simulink model "2.LC vs. LCL"  (R2022b)
settings: Solver=ode23tb  StartTime=0.0  StopTime=0.06  RelTol=1e-3
libraries: spsCurrentMeasurementLib x18, spsSeriesRLCBranchLib x17, spsIGBTDiodeLib x12, spsabctodq0Lib x4, spsDCVoltageSourceLib x2, spsGroundLib x2, spsThreePhaseSeriesRLCLoadLib x2, spsThreePhaseTransformerTwoWindingsLib x2, spsThreePhaseVIMeasurementLib x2, spsSVPWMGenerator2LevelLib x1, spsabctoAlphaBetaZeroLib x1, spspowerguiLib x1
settings Model: Creator=Mushrif  LastModifiedBy=Mushrif

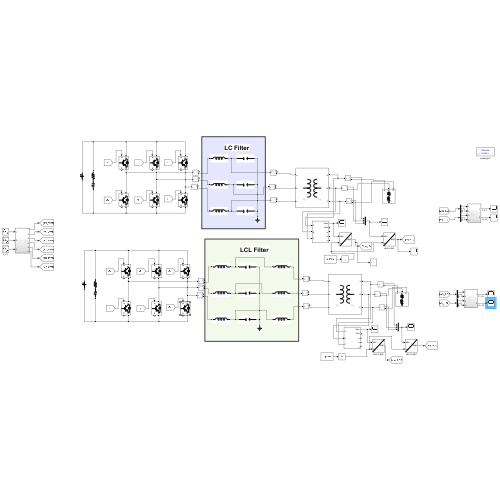
[thumbnail: Simulink's stored preview of the top-level diagram]
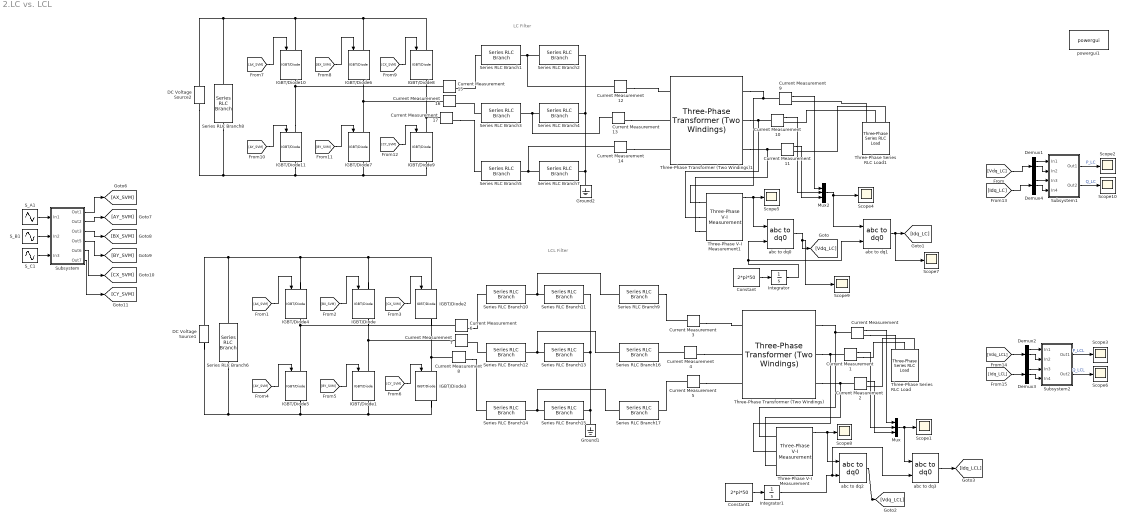
== system 2.LC vs. LCL ==
  note: LCL Filter
  note: LC Filter
  Constant : Constant  Value=2*pi*50
  Constant1 : Constant  Value=2*pi*50
  Current Measurement{,1..17} (18 alike) : spsCurrentMeasurementLib/Current Measurement  PhasorSimulation=off  OutputType=Complex  PSBequivalent=0
  DC Voltage Source1 : spsDCVoltageSourceLib/DC Voltage Source  Amplitude=78  Measurements=None
  DC Voltage Source2 : spsDCVoltageSourceLib/DC Voltage Source  Amplitude=82  Measurements=None
  Demux{1..4} (4 alike) : Demux  Outputs=3
  Ground1 : spsGroundLib/Ground  LConnTagsString=a
  Ground2 : spsGroundLib/Ground  LConnTagsString=a
  IGBT/Diode{,1..11} (12 alike) : spsIGBTDiodeLib/IGBT//Diode  Ron=1e-3  Rs=1e5  Cs=inf  Measurements=on
  Integrator : Integrator
  Integrator1 : Integrator
  Mux : Mux  Inputs=3
  Mux2 : Mux  Inputs=3
  S_A1 : Sin  Amplitude=0.9  Frequency=2*pi*50  SampleTime=0
  S_B1 : Sin  Amplitude=0.9  Frequency=2*pi*50  Phase=-2*pi/3  SampleTime=0
  S_C1 : Sin  Amplitude=0.9  Frequency=2*pi*50  Phase=2*pi/3  SampleTime=0
  Scope{1..10} (10 alike) : Scope
  Series RLC Branch{1,3,5,9,16..17} (6 alike) : spsSeriesRLCBranchLib/Series RLC Branch  LConnTagsString=__new0  RConnTagsString=__new0  BranchType=L  Resistance=2.2  Inductance=250e-6  SetiL0=off  InitialCurrent=0  Capacitance=1e-6  Setx0=off  InitialVoltage=0  Measurements=None
  Series RLC Branch10 : spsSeriesRLCBranchLib/Series RLC Branch  LConnTagsString=__new0  RConnTagsString=__new0  BranchType=L  Resistance=2.2  Inductance=100e-9  SetiL0=off  InitialCurrent=0  Capacitance=1e-6  Setx0=off  InitialVoltage=0  Measurements=None
  Series RLC Branch11 : spsSeriesRLCBranchLib/Series RLC Branch  LConnTagsString=__new0  RConnTagsString=__new0  BranchType=C  Resistance=1  Inductance=1e-3  SetiL0=off  InitialCurrent=0  Capacitance=40e-3  Setx0=off  InitialVoltage=0  Measurements=None
  Series RLC Branch12 : spsSeriesRLCBranchLib/Series RLC Branch  LConnTagsString=__new0  RConnTagsString=__new0  BranchType=L  Resistance=2.2  Inductance=100e-9  SetiL0=off  InitialCurrent=0  Capacitance=1e-6  Setx0=off  InitialVoltage=0  Measurements=None
  Series RLC Branch13 : spsSeriesRLCBranchLib/Series RLC Branch  LConnTagsString=__new0  RConnTagsString=__new0  BranchType=C  Resistance=1  Inductance=1e-3  SetiL0=off  InitialCurrent=0  Capacitance=40e-3  Setx0=off  InitialVoltage=0  Measurements=None
  Series RLC Branch14 : spsSeriesRLCBranchLib/Series RLC Branch  LConnTagsString=__new0  RConnTagsString=__new0  BranchType=L  Resistance=2.2  Inductance=100e-9  SetiL0=off  InitialCurrent=0  Capacitance=1e-6  Setx0=off  InitialVoltage=0  Measurements=None
  Series RLC Branch15 : spsSeriesRLCBranchLib/Series RLC Branch  LConnTagsString=__new0  RConnTagsString=__new0  BranchType=C  Resistance=1  Inductance=1e-3  SetiL0=off  InitialCurrent=0  Capacitance=40e-3  Setx0=off  InitialVoltage=0  Measurements=None
  Series RLC Branch2 : spsSeriesRLCBranchLib/Series RLC Branch  LConnTagsString=__new0  RConnTagsString=__new0  BranchType=C  Resistance=1  Inductance=1e-3  SetiL0=off  InitialCurrent=0  Capacitance=40e-6  Setx0=off  InitialVoltage=0  Measurements=None
  Series RLC Branch4 : spsSeriesRLCBranchLib/Series RLC Branch  LConnTagsString=__new0  RConnTagsString=__new0  BranchType=C  Resistance=1  Inductance=1e-3  SetiL0=off  InitialCurrent=0  Capacitance=40e-6  Setx0=off  InitialVoltage=0  Measurements=None
  Series RLC Branch6 : spsSeriesRLCBranchLib/Series RLC Branch  LConnTagsString=__new0  RConnTagsString=__new0  BranchType=RC  Resistance=0.02  Inductance=1e-3  SetiL0=off  InitialCurrent=0  Capacitance=0.001  Setx0=off  InitialVoltage=0  Measurements=None
  Series RLC Branch7 : spsSeriesRLCBranchLib/Series RLC Branch  LConnTagsString=__new0  RConnTagsString=__new0  BranchType=C  Resistance=1  Inductance=1e-3  SetiL0=off  InitialCurrent=0  Capacitance=40e-6  Setx0=off  InitialVoltage=0  Measurements=None
  Series RLC Branch8 : spsSeriesRLCBranchLib/Series RLC Branch  LConnTagsString=__new0  RConnTagsString=__new0  BranchType=RC  Resistance=0.02  Inductance=1e-3  SetiL0=off  InitialCurrent=0  Capacitance=0.001  Setx0=off  InitialVoltage=0  Measurements=None
  Subsystem : Subsystem
  Subsystem1 : Subsystem
  Subsystem2 : Subsystem
  Three-Phase Series RLC Load : spsThreePhaseSeriesRLCLoadLib/Three-Phase Series RLC Load  LConnTagsString=A|B|C  Configuration=Y (grounded)  NominalVoltage=400  Vabc=[1e3 1e3 1e3]  Vabcp=[1e3 1e3 1e3]  NominalFrequency=50  UnbalancedPower=off  ActivePower=1500  InductivePower=100  CapacitivePower=0  Pabc=[10e3 9e3 11e3]  QLabc=[100 90 110]  QCabc=[100 90 110]  Pabcp=[10e3 9e3 11e3]  QLabcp=[100 90 110]  QCabcp=[100 90 110]  Measurements=None  LoadType=constant Z
  Three-Phase Series RLC Load1 : spsThreePhaseSeriesRLCLoadLib/Three-Phase Series RLC Load  LConnTagsString=A|B|C  Configuration=Y (grounded)  NominalVoltage=400  Vabc=[1e3 1e3 1e3]  Vabcp=[1e3 1e3 1e3]  NominalFrequency=50  UnbalancedPower=off  ActivePower=1500  InductivePower=100  CapacitivePower=0  Pabc=[10e3 9e3 11e3]  QLabc=[100 90 110]  QCabc=[100 90 110]  Pabcp=[10e3 9e3 11e3]  QLabcp=[100 90 110]  QCabcp=[100 90 110]  Measurements=None  LoadType=constant Z
  Three-Phase Transformer (Two Windings) : spsThreePhaseTransformerTwoWindingsLib/Three-Phase Transformer (Two Windings)  Winding1Connection=Yg  Winding2Connection=Yg  CoreType=Three single-phase transformers  SetSaturation=off  Hysteresis=off  DataFile='hysteresis'  SetInitialFlux=off  Measurements=None  UNITS=SI  NominalPower=[ 1900 , 50 ]  Winding1=[415 0.0001 0.0001]  Winding2=[47 0.0001 0.0001]  Rm=45322  Lm=144.27  L0=0.5  Saturation=[0 0;0.0089716 1.2943;3.7382 1.6394]  InitialFluxes=[ 0.8 , -0.8 , 0.7 ]  BreakLoop=off  DiscreteSolver=Trapezoidal iterative  DataType=on  TransfoNumber=1
  Three-Phase Transformer (Two Windings)1 : spsThreePhaseTransformerTwoWindingsLib/Three-Phase Transformer (Two Windings)  Winding1Connection=Yg  Winding2Connection=Yg  CoreType=Three single-phase transformers  SetSaturation=off  Hysteresis=off  DataFile='hysteresis'  SetInitialFlux=off  Measurements=None  UNITS=SI  NominalPower=[ 1900 , 50 ]  Winding1=[415 0.0001 0.0001]  Winding2=[47 0.0001 0.0001]  Rm=45322  Lm=144.27  L0=0.5  Saturation=[0 0;0.0089716 1.2943;3.7382 1.6394]  InitialFluxes=[ 0.8 , -0.8 , 0.7 ]  BreakLoop=off  DiscreteSolver=Trapezoidal iterative  DataType=on  TransfoNumber=1
  Three-Phase V-I Measurement : spsThreePhaseVIMeasurementLib/Three-Phase V-I Measurement  VoltageMeasurement=phase-to-phase  SetLabelV=off  LabelV=Vabc  Vpu=off  VpuLL=off  CurrentMeasurement=yes  SetLabelI=off  LabelI=Iabc  Ipu=off  Pbase=100e6  Vbase=500e3  OutputType=Complex  PhasorSimulation=off  PSBequivalent=0
  Three-Phase V-I Measurement1 : spsThreePhaseVIMeasurementLib/Three-Phase V-I Measurement  VoltageMeasurement=phase-to-phase  SetLabelV=off  LabelV=Vabc  Vpu=off  VpuLL=off  CurrentMeasurement=yes  SetLabelI=off  LabelI=Iabc  Ipu=off  Pbase=100e6  Vbase=500e3  OutputType=Complex  PhasorSimulation=off  PSBequivalent=0
  abc to dq{0..3} (4 alike) : spsabctodq0Lib/abc to dq0  Alignment=90 degrees behind phase A axis
  powergui1 : spspowerguiLib/powergui  Priority=1  SimulationMode=Discrete  SampleTime=5e-8  frequency=60  Iterations=50  frequencyindice=0  Pbase=100e6  ErrMax=1e-4  UnitsV=kV  UnitsW=MW  buscounter=0  FunctionMessages=off  echomessages=off  EnableUseOfTLC=off  CurrentSourceSwitches=off  DisableSnubberDevices=off  DisableRonSwitches=off  DisableVfSwitches=off  DisplayEquations=off  AutomaticDiscreteSolvers=off  SolverType=Tustin/Backward Euler (TBE)  Interpol=off  ExternalGateDelay=off  methode=off  Ts=100  x0status=blocks  SPID=on  SwTol=0  HookPort=off  NonlinearTolerance=1e-4  nMaxIteration=100  ContinueOnMaxIteration=off  RestoreLinks=warning  ResistiveCurrentMeasurement=off  Frange=[0:2:500]  Ylog=off  Xlog=on  ShowGrid=off  save=off  variable=ZData  structure=0  ZoomFFT=off  StartTime=0.0  cycles=1  DisplayStyle=1  fundamental=60  FreqAxis=off  MaxFrequency=1000  frequencyindicesteady=1  RmsSteady=1  display=off
  wires:
  Three-Phase V-I Measurement/1 -> abc to dq2/1, Scope8/1
  [AX_SVM] -> IGBT/Diode4/1
  [AY_SVM] -> IGBT/Diode5/1
  [BX_SVM] -> IGBT/Diode/1
  [BY_SVM] -> IGBT/Diode1/1
  [CX_SVM] -> IGBT/Diode2/1
  [CY_SVM] -> IGBT/Diode3/1
  Current Measurement/1 -> Mux/1
  Current Measurement1/1 -> Mux/2
  Current Measurement2/1 -> Mux/3
  Mux/1 -> abc to dq3/1, Scope1/1
  Current Measurement11/1 -> Mux2/3
  Current Measurement10/1 -> Mux2/2
  Current Measurement9/1 -> Mux2/1
  [AY_SVM] -> IGBT/Diode11/1
  [AX_SVM] -> IGBT/Diode10/1
  [CY_SVM] -> IGBT/Diode9/1
  [CX_SVM] -> IGBT/Diode8/1
  [BY_SVM] -> IGBT/Diode7/1
  [BX_SVM] -> IGBT/Diode6/1
  Mux2/1 -> abc to dq1/1, Scope4/1
  S_A1/1 -> Subsystem/1(In1)
  S_B1/1 -> Subsystem/2(In2)
  S_C1/1 -> Subsystem/3(In3)
  Subsystem/1(Out1) -> [AX_SVM]
  Subsystem/2(Out2) -> [AY_SVM]
  Subsystem/3(Out3) -> [BX_SVM]
  Subsystem/4(Out5) -> [BY_SVM]
  Subsystem/5(Out6) -> [CX_SVM]
  Subsystem/6(Out7) -> [CY_SVM]
  Three-Phase V-I Measurement1/1 -> abc to dq0/1, Scope5/1
  abc to dq0/1 -> Scope9/1, [Vdq_LC]
  abc to dq1/1 -> Scope7/1, [Idq_LC]
  abc to dq2/1 -> [Vdq_LCL]
  abc to dq3/1 -> [Idq_LCL]
  Subsystem2/1(Out1) -> Scope3/1  "P_LCL"
  Demux2/2 -> Subsystem2/2(In2)
  [Vdq_LCL] -> Demux2/1
  Demux3/2 -> Subsystem2/4(In4)
  Demux3/1 -> Subsystem2/3(In3)
  Demux2/1 -> Subsystem2/1(In1)
  Subsystem2/2(Out2) -> Scope6/1  "Q_LCL"
  [Idq_LCL] -> Demux3/1
  Constant/1 -> Integrator/1
  Integrator/1 -> abc to dq1/2, abc to dq0/2
  Constant1/1 -> Integrator1/1
  Integrator1/1 -> abc to dq3/2, abc to dq2/2
  [Idq_LC] -> Demux4/1
  Subsystem1/2(Out2) -> Scope10/1  "Q_LC"
  Demux1/1 -> Subsystem1/1(In1)
  Demux4/1 -> Subsystem1/3(In3)
  Demux1/2 -> Subsystem1/2(In2)
  Demux4/2 -> Subsystem1/4(In4)
  [Vdq_LC] -> Demux1/1
  Subsystem1/1(Out1) -> Scope2/1  "P_LC"
  connections:
  IGBT/Diode/LConn1 -- IGBT/Diode2/LConn1 -- Series RLC Branch6/LConn1 -- DC Voltage Source1/RConn1 -- IGBT/Diode4/LConn1
  DC Voltage Source1/LConn1 -- Series RLC Branch6/RConn1 -- IGBT/Diode5/RConn1 -- IGBT/Diode3/RConn1 -- IGBT/Diode1/RConn1
  IGBT/Diode/RConn1 -- IGBT/Diode1/LConn1 -- Current Measurement7/LConn1
  IGBT/Diode2/RConn1 -- IGBT/Diode3/LConn1 -- Current Measurement8/LConn1
  Three-Phase Transformer (Two Windings)/LConn2 -- Current Measurement1/LConn1 -- Three-Phase V-I Measurement/LConn2
  IGBT/Diode4/RConn1 -- Current Measurement6/LConn1 -- IGBT/Diode5/LConn1
  Series RLC Branch13/LConn1 -- Series RLC Branch16/LConn1 -- Series RLC Branch12/RConn1
  Series RLC Branch15/LConn1 -- Series RLC Branch17/LConn1 -- Series RLC Branch14/RConn1
  Series RLC Branch11/LConn1 -- Series RLC Branch9/LConn1 -- Series RLC Branch10/RConn1
  Series RLC Branch11/RConn1 -- Series RLC Branch15/RConn1 -- Ground1/LConn1 -- Series RLC Branch13/RConn1
  Three-Phase Transformer (Two Windings)/LConn1 -- Current Measurement/LConn1 -- Three-Phase V-I Measurement/LConn1
  Three-Phase Transformer (Two Windings)/LConn3 -- Current Measurement2/LConn1 -- Three-Phase V-I Measurement/LConn3
  Current Measurement3/RConn1 -- Three-Phase Transformer (Two Windings)/RConn1
  Current Measurement4/RConn1 -- Three-Phase Transformer (Two Windings)/RConn2
  Current Measurement5/RConn1 -- Three-Phase Transformer (Two Windings)/RConn3
  Current Measurement6/RConn1 -- Series RLC Branch10/LConn1
  Series RLC Branch12/LConn1 -- Current Measurement7/RConn1
  Current Measurement8/RConn1 -- Series RLC Branch14/LConn1
  Current Measurement/RConn1 -- Three-Phase Series RLC Load/LConn1
  Current Measurement1/RConn1 -- Three-Phase Series RLC Load/LConn2
  Three-Phase Series RLC Load/LConn3 -- Current Measurement2/RConn1
  Three-Phase V-I Measurement1/LConn3 -- Three-Phase Transformer (Two Windings)1/LConn3 -- Current Measurement11/LConn1
  Series RLC Branch5/RConn1 -- Series RLC Branch7/LConn1 -- Current Measurement14/LConn1
  Series RLC Branch1/RConn1 -- Series RLC Branch2/LConn1 -- Current Measurement12/LConn1
  IGBT/Diode11/LConn1 -- IGBT/Diode10/RConn1 -- Current Measurement15/LConn1
  IGBT/Diode10/LConn1 -- IGBT/Diode6/LConn1 -- IGBT/Diode8/LConn1 -- Series RLC Branch8/LConn1 -- DC Voltage Source2/RConn1
  Current Measurement16/LConn1 -- IGBT/Diode6/RConn1 -- IGBT/Diode7/LConn1
  Series RLC Branch4/LConn1 -- Current Measurement13/LConn1 -- Series RLC Branch3/RConn1
  IGBT/Diode7/RConn1 -- IGBT/Diode9/RConn1 -- DC Voltage Source2/LConn1 -- Series RLC Branch8/RConn1 -- IGBT/Diode11/RConn1
  Three-Phase V-I Measurement1/LConn2 -- Three-Phase Transformer (Two Windings)1/LConn2 -- Current Measurement10/LConn1
  Series RLC Branch4/RConn1 -- Series RLC Branch7/RConn1 -- Ground2/LConn1 -- Series RLC Branch2/RConn1
  Three-Phase V-I Measurement1/LConn1 -- Three-Phase Transformer (Two Windings)1/LConn1 -- Current Measurement9/LConn1
  Current Measurement17/LConn1 -- IGBT/Diode8/RConn1 -- IGBT/Diode9/LConn1
  Three-Phase Series RLC Load1/LConn3 -- Current Measurement11/RConn1
  Three-Phase Series RLC Load1/LConn2 -- Current Measurement10/RConn1
  Current Measurement15/RConn1 -- Series RLC Branch1/LConn1
  Current Measurement17/RConn1 -- Series RLC Branch5/LConn1
  Three-Phase Series RLC Load1/LConn1 -- Current Measurement9/RConn1
  Current Measurement12/RConn1 -- Three-Phase Transformer (Two Windings)1/RConn1
  Series RLC Branch3/LConn1 -- Current Measurement16/RConn1
  Current Measurement14/RConn1 -- Three-Phase Transformer (Two Windings)1/RConn3
  Current Measurement13/RConn1 -- Three-Phase Transformer (Two Windings)1/RConn2
  Series RLC Branch9/RConn1 -- Current Measurement3/LConn1
  Current Measurement4/LConn1 -- Series RLC Branch16/RConn1
  Current Measurement5/LConn1 -- Series RLC Branch17/RConn1

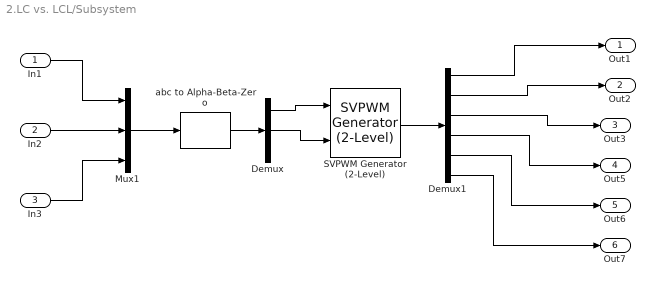
== system 2.LC vs. LCL/Subsystem ==
  In1 : Inport
  In2 : Inport  Port=2
  In3 : Inport  Port=3
  Demux : Demux  Outputs=3
  Demux1 : Demux  Outputs=6
  Mux1 : Mux  Inputs=3
  SVPWM Generator (2-Level) : spsSVPWMGenerator2LevelLib/SVPWM Generator (2-Level)  InputType=alpha-beta components  SwitchingPattern=Pattern #1  Fc=20000  ParUref=[0.8 -30 50]  Ts=0
  abc to Alpha-Beta-Zero : spsabctoAlphaBetaZeroLib/abc to Alpha-Beta-Zero
  Out1 : Outport
  Out2 : Outport  Port=2
  Out3 : Outport  Port=3
  Out5 : Outport  Port=4
  Out6 : Outport  Port=5
  Out7 : Outport  Port=6
  wires:
  Demux1/4 -> Out5/1
  Mux1/1 -> abc to Alpha-Beta-Zero/1
  Demux1/3 -> Out3/1
  abc to Alpha-Beta-Zero/1 -> Demux/1
  Demux/2 -> SVPWM Generator (2-Level)/2
  Demux1/1 -> Out1/1
  Demux1/6 -> Out7/1
  In3/1 -> Mux1/3
  Demux/1 -> SVPWM Generator (2-Level)/1
  SVPWM Generator (2-Level)/1 -> Demux1/1
  Demux1/2 -> Out2/1
  In1/1 -> Mux1/1
  In2/1 -> Mux1/2
  Demux1/5 -> Out6/1

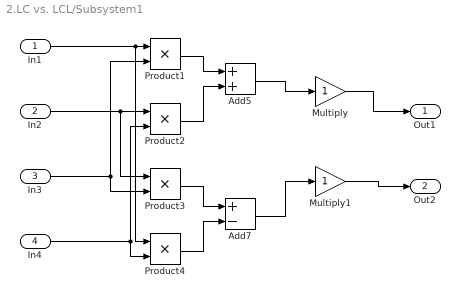
== system 2.LC vs. LCL/Subsystem1 ==
  In1 : Inport
  In2 : Inport  Port=2
  In3 : Inport  Port=3
  In4 : Inport  Port=4
  Add5 : Sum
  Add7 : Sum  Inputs=+-
  Multiply : Gain
  Multiply1 : Gain
  Product{1..4} (4 alike) : Product
  Out1 : Outport
  Out2 : Outport  Port=2
  wires:
  Product4/1 -> Add7/2
  In4/1 -> Product4/2, Product2/2
  Product1/1 -> Add5/1
  Product2/1 -> Add5/2
  In3/1 -> Product3/2, Product1/2
  In2/1 -> Product3/1, Product2/1
  Product3/1 -> Add7/1
  In1/1 -> Product4/1, Product1/1
  Add5/1 -> Multiply/1
  Add7/1 -> Multiply1/1
  Multiply/1 -> Out1/1
  Multiply1/1 -> Out2/1

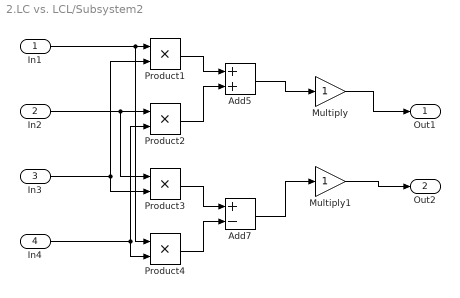
== system 2.LC vs. LCL/Subsystem2 ==
  In1 : Inport
  In2 : Inport  Port=2
  In3 : Inport  Port=3
  In4 : Inport  Port=4
  Add5 : Sum
  Add7 : Sum  Inputs=+-
  Multiply : Gain
  Multiply1 : Gain
  Product{1..4} (4 alike) : Product
  Out1 : Outport
  Out2 : Outport  Port=2
  wires:
  Product4/1 -> Add7/2
  In4/1 -> Product4/2, Product2/2
  Product1/1 -> Add5/1
  Product2/1 -> Add5/2
  In3/1 -> Product3/2, Product1/2
  In2/1 -> Product3/1, Product2/1
  Product3/1 -> Add7/1
  In1/1 -> Product4/1, Product1/1
  Add5/1 -> Multiply/1
  Add7/1 -> Multiply1/1
  Multiply/1 -> Out1/1
  Multiply1/1 -> Out2/1
